simulink model "IndicatorBoard"  (R2023a)
settings: Solver=VariableStepAuto  StartTime=0.0  StopTime=10.0  RelTol=1e-3
libraries: simulink x2
settings Model: Creator=lucas  LastModifiedBy=lucas

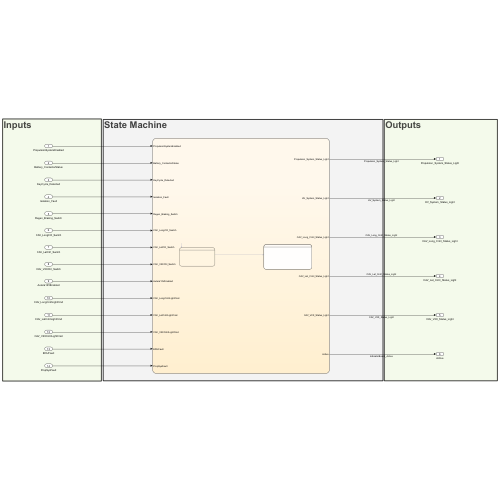
[thumbnail: Simulink's stored preview of the top-level diagram]
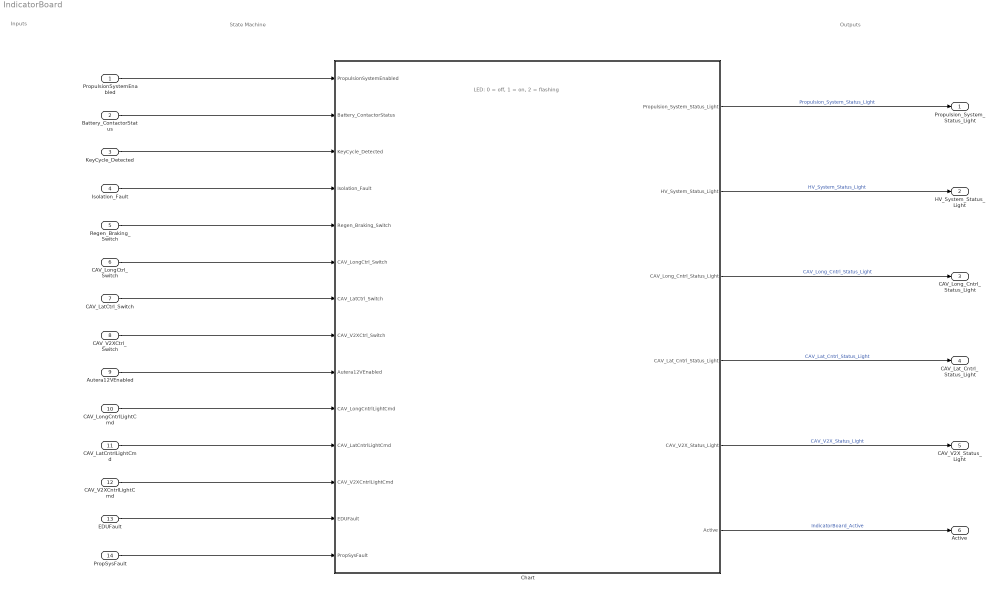
== system IndicatorBoard ==
  note: Inputs
  note: LED: 0 = off, 1 = on, 2 = flashing
  note: Outputs
  note: State Machine
  PropulsionSystemEnabled : Inport
  Battery_ContactorStatus : Inport  Port=2
  KeyCycle_Detected : Inport  Port=3
  Isolation_Fault : Inport  Port=4
  Regen_Braking_Switch : Inport  Port=5
  CAV_LongCtrl_Switch : Inport  Port=6
  CAV_LatCtrl_Switch : Inport  Port=7
  CAV_V2XCtrl_Switch : Inport  Port=8
  Autera12VEnabled : Inport  Port=9
  CAV_LongCntrlLightCmd : Inport  Port=10
  CAV_LatCntrlLightCmd : Inport  Port=11
  CAV_V2XCntrlLightCmd : Inport  Port=12
  EDUFault : Inport  Port=13
  PropSysFault : Inport  Port=14
  Chart : Stateflow chart  TreatAsAtomicUnit=on
  Propulsion_System_Status_Light : Outport
  HV_System_Status_Light : Outport  Port=2
  CAV_Long_Cntrl_Status_Light : Outport  Port=3
  CAV_Lat_Cntrl_Status_Light : Outport  Port=4
  CAV_V2X_Status_Light : Outport  Port=5
  Active : Outport  Port=6
  wires:
  Chart/1(Propulsion_System_Status_Light) -> Propulsion_System_Status_Light/1  "Propulsion_System_Status_Light"
  KeyCycle_Detected/1 -> Chart/3(KeyCycle_Detected)
  Chart/2(HV_System_Status_Light) -> HV_System_Status_Light/1  "HV_System_Status_Light"
  Chart/5(CAV_V2X_Status_Light) -> CAV_V2X_Status_Light/1  "CAV_V2X_Status_Light"
  PropulsionSystemEnabled/1 -> Chart/1(PropulsionSystemEnabled)
  Chart/4(CAV_Lat_Cntrl_Status_Light) -> CAV_Lat_Cntrl_Status_Light/1  "CAV_Lat_Cntrl_Status_Light"
  Chart/3(CAV_Long_Cntrl_Status_Light) -> CAV_Long_Cntrl_Status_Light/1  "CAV_Long_Cntrl_Status_Light"
  Battery_ContactorStatus/1 -> Chart/2(Battery_ContactorStatus)
  Autera12VEnabled/1 -> Chart/9(Autera12VEnabled)
  Isolation_Fault/1 -> Chart/4(Isolation_Fault)
  Regen_Braking_Switch/1 -> Chart/5(Regen_Braking_Switch)
  CAV_LongCtrl_Switch/1 -> Chart/6(CAV_LongCtrl_Switch)
  CAV_LatCtrl_Switch/1 -> Chart/7(CAV_LatCtrl_Switch)
  CAV_V2XCtrl_Switch/1 -> Chart/8(CAV_V2XCtrl_Switch)
  CAV_LongCntrlLightCmd/1 -> Chart/10(CAV_LongCntrlLightCmd)
  EDUFault/1 -> Chart/13(EDUFault)
  CAV_LatCntrlLightCmd/1 -> Chart/11(CAV_LatCntrlLightCmd)
  CAV_V2XCntrlLightCmd/1 -> Chart/12(CAV_V2XCntrlLightCmd)
  PropSysFault/1 -> Chart/14(PropSysFault)
  Chart/6(Active) -> Active/1  "IndicatorBoard_Active"

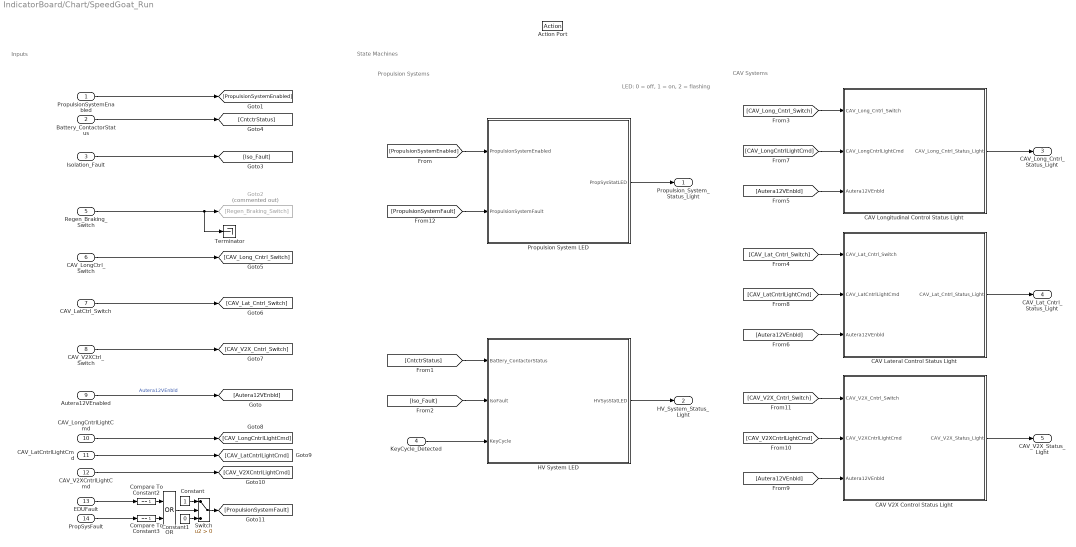
== system IndicatorBoard/Chart/SpeedGoat_Run ==
  note: LED: 0 = off, 1 = on, 2 = flashing
  note: Inputs
  note: State Machines
  note: Propulsion Systems
  note: CAV Systems
  PropulsionSystemEnabled : Inport
  Battery_ContactorStatus : Inport  Port=2
  Isolation_Fault : Inport  Port=3
  KeyCycle_Detected : Inport  Port=4
  Regen_Braking_Switch : Inport  Port=5
  CAV_LongCtrl_Switch : Inport  Port=6
  CAV_LatCtrl_Switch : Inport  Port=7
  CAV_V2XCtrl_Switch : Inport  Port=8
  Autera12VEnabled : Inport  Port=9
  CAV_LongCntrlLightCmd : Inport  Port=10
  CAV_LatCntrlLightCmd : Inport  Port=11
  CAV_V2XCntrlLightCmd : Inport  Port=12
  EDUFault : Inport  Port=13
  PropSysFault : Inport  Port=14
  Action Port : ActionPort
      settings: CopyFcn=Stateflow.SLINSF.SimulinkMan.removeBlockPreDeleteFcn  PreDeleteFcn=Stateflow.SLINSF.SimulinkMan.unsafePredeleteFcn
  CAV Lateral Control Status Light : Stateflow chart  TreatAsAtomicUnit=on
  CAV Longitudinal Control Status Light : Stateflow chart  TreatAsAtomicUnit=on
  CAV V2X Control Status Light : Stateflow chart  TreatAsAtomicUnit=on
  Compare To Constant2 : simulink/Logic and Bit Operations/Compare To Constant  relop===  const=1  OutDataTypeStr=boolean
  Compare To Constant3 : simulink/Logic and Bit Operations/Compare To Constant  relop===  const=1  OutDataTypeStr=boolean
  Constant : Constant
  Constant1 : Constant  Value=0
  Goto2 : Goto  Commented=on  GotoTag=Regen_Braking_Switch
  HV System LED : Stateflow chart  TreatAsAtomicUnit=on
  OR : Logic  Operator=OR  AllPortsSameDT=off  OutDataTypeStr=boolean
  Propulsion System LED : Stateflow chart  TreatAsAtomicUnit=on
  Switch : Switch  Criteria=u2 > Threshold  SaturateOnIntegerOverflow=off  InputSameDT=off
  Terminator : Terminator
  Propulsion_System_Status_Light : Outport
  HV_System_Status_Light : Outport  Port=2
  CAV_Long_Cntrl_Status_Light : Outport  Port=3
  CAV_Lat_Cntrl_Status_Light : Outport  Port=4
  CAV_V2X_Status_Light : Outport  Port=5
  wires:
  KeyCycle_Detected/1 -> HV System LED/3(KeyCycle)
  CAV V2X Control Status Light/1(CAV_V2X_Status_Light) -> CAV_V2X_Status_Light/1
  Constant1/1 -> Switch/3
  Constant/1 -> Switch/1
  Switch/1 -> [PropulsionSystemFault]
  [PropulsionSystemFault] -> Propulsion System LED/2(PropulsionSystemFault)
  OR/1 -> Switch/2
  Compare To Constant3/1 -> OR/2
  Compare To Constant2/1 -> OR/1
  PropSysFault/1 -> Compare To Constant3/1
  EDUFault/1 -> Compare To Constant2/1
  [CAV_V2X_Cntrl_Switch] -> CAV V2X Control Status Light/1(CAV_V2X_Cntrl_Switch)
  [CAV_V2XCntrlLightCmd] -> CAV V2X Control Status Light/2(CAV_V2XCntrlLightCmd)
  [Autera12VEnbld] -> CAV V2X Control Status Light/3(Autera12VEnbld)
  [Autera12VEnbld] -> CAV Lateral Control Status Light/3(Autera12VEnbld)
  [CAV_LatCntrlLightCmd] -> CAV Lateral Control Status Light/2(CAV_LatCntrlLightCmd)
  [CAV_Lat_Cntrl_Switch] -> CAV Lateral Control Status Light/1(CAV_Lat_Cntrl_Switch)
  [CAV_LongCntrlLightCmd] -> CAV Longitudinal Control Status Light/2(CAV_LongCntrlLightCmd)
  CAV_V2XCntrlLightCmd/1 -> [CAV_V2XCntrlLightCmd]
  CAV_LatCntrlLightCmd/1 -> [CAV_LatCntrlLightCmd]
  CAV_LongCntrlLightCmd/1 -> [CAV_LongCntrlLightCmd]
  [CAV_Long_Cntrl_Switch] -> CAV Longitudinal Control Status Light/1(CAV_Long_Cntrl_Switch)
  [Autera12VEnbld] -> CAV Longitudinal Control Status Light/3(Autera12VEnbld)
  CAV Longitudinal Control Status Light/1(CAV_Long_Cntrl_Status_Light) -> CAV_Long_Cntrl_Status_Light/1
  CAV Lateral Control Status Light/1(CAV_Lat_Cntrl_Status_Light) -> CAV_Lat_Cntrl_Status_Light/1
  HV System LED/1(HVSysStatLED) -> HV_System_Status_Light/1
  Propulsion System LED/1(PropSysStatLED) -> Propulsion_System_Status_Light/1
  [Iso_Fault] -> HV System LED/2(IsoFault)
  [CntctrStatus] -> HV System LED/1(Battery_ContactorStatus)
  [PropulsionSystemEnabled] -> Propulsion System LED/1(PropulsionSystemEnabled)
  CAV_V2XCtrl_Switch/1 -> [CAV_V2X_Cntrl_Switch]
  CAV_LatCtrl_Switch/1 -> [CAV_Lat_Cntrl_Switch]
  CAV_LongCtrl_Switch/1 -> [CAV_Long_Cntrl_Switch]
  Regen_Braking_Switch/1 -> Terminator/1, Goto2/1
  Autera12VEnabled/1 -> [Autera12VEnbld]  "Autera12VEnbld"
  Battery_ContactorStatus/1 -> [CntctrStatus]
  PropulsionSystemEnabled/1 -> [PropulsionSystemEnabled]
  Isolation_Fault/1 -> [Iso_Fault]

== stateflow chart IndicatorBoard/Chart ==
  state SpeedGoat_Run
  state SpeedGoat_Startup
    state On_Off [group]
      state All_Off
        entry:
        CAV_Lat_Cntrl_Status_Light = 0;
        CAV_Long_Cntrl_Status_Light = 0;
        CAV_V2X_Status_Light = 0;
        HV_System_Status_Light = 0;
        Propulsion_System_Status_Light = 0;
      state All_On
        entry:
        CAV_Lat_Cntrl_Status_Light = 1;
        CAV_Long_Cntrl_Status_Light = 1;
        CAV_V2X_Status_Light = 1;
        HV_System_Status_Light = 1;
        Propulsion_System_Status_Light = 1;
      state All_Off1
        entry:
        CAV_Lat_Cntrl_Status_Light = 0;
        CAV_Long_Cntrl_Status_Light = 0;
        CAV_V2X_Status_Light = 0;
        HV_System_Status_Light = 0;
        Propulsion_System_Status_Light = 0;
      state All_On1
        entry:
        CAV_Lat_Cntrl_Status_Light = 1;
        CAV_Long_Cntrl_Status_Light = 1;
        CAV_V2X_Status_Light = 1;
        HV_System_Status_Light = 1;
        Propulsion_System_Status_Light = 1;
      state All_Off2
        entry:
        CAV_Lat_Cntrl_Status_Light = 0;
        CAV_Long_Cntrl_Status_Light = 0;
        CAV_V2X_Status_Light = 0;
        HV_System_Status_Light = 0;
        Propulsion_System_Status_Light = 0;
      state All_On2
        entry:
        CAV_Lat_Cntrl_Status_Light = 1;
        CAV_Long_Cntrl_Status_Light = 1;
        CAV_V2X_Status_Light = 1;
        HV_System_Status_Light = 1;
        Propulsion_System_Status_Light = 1;
      state All_Off3
        entry:
        CAV_Lat_Cntrl_Status_Light = 0;
        CAV_Long_Cntrl_Status_Light = 0;
        CAV_V2X_Status_Light = 0;
        HV_System_Status_Light = 0;
        Propulsion_System_Status_Light = 0;
      (default) -> All_Off
      All_On -> All_Off1 : after(0.2,sec)
      All_Off1 -> All_On1 : after(0.2,sec)
      All_On1 -> All_Off2 : after(0.2,sec)
      All_On2 -> All_Off3 : after(0.2,sec)
      All_Off2 -> All_On2 : after(0.2,sec)
      All_Off -> All_On : after(0.2,sec)
    state Side_To_Side [group]
      state LED2_2
        entry:
        CAV_Lat_Cntrl_Status_Light = 0;
        CAV_Long_Cntrl_Status_Light = 0;
        CAV_V2X_Status_Light = 0;
        HV_System_Status_Light = 1;
        Propulsion_System_Status_Light = 0;
      state LED1_1
        entry:
        CAV_Lat_Cntrl_Status_Light = 0;
        CAV_Long_Cntrl_Status_Light = 0;
        CAV_V2X_Status_Light = 0;
        HV_System_Status_Light = 0;
        Propulsion_System_Status_Light = 1;
      state LED1_2
        entry:
        CAV_Lat_Cntrl_Status_Light = 0;
        CAV_Long_Cntrl_Status_Light = 0;
        CAV_V2X_Status_Light = 0;
        HV_System_Status_Light = 0;
        Propulsion_System_Status_Light = 1;
      state LED1_3
        entry:
        CAV_Lat_Cntrl_Status_Light = 0;
        CAV_Long_Cntrl_Status_Light = 0;
        CAV_V2X_Status_Light = 0;
        HV_System_Status_Light = 0;
        Propulsion_System_Status_Light = 1;
      state LED1_4
        entry:
        CAV_Lat_Cntrl_Status_Light = 0;
        CAV_Long_Cntrl_Status_Light = 0;
        CAV_V2X_Status_Light = 0;
        HV_System_Status_Light = 0;
        Propulsion_System_Status_Light = 1;
      state LED2_6
        entry:
        CAV_Lat_Cntrl_Status_Light = 0;
        CAV_Long_Cntrl_Status_Light = 0;
        CAV_V2X_Status_Light = 0;
        HV_System_Status_Light = 1;
        Propulsion_System_Status_Light = 0;
      state LED2_4
        entry:
        CAV_Lat_Cntrl_Status_Light = 0;
        CAV_Long_Cntrl_Status_Light = 0;
        CAV_V2X_Status_Light = 0;
        HV_System_Status_Light = 1;
        Propulsion_System_Status_Light = 0;
      state LED3_2
        entry:
        CAV_Lat_Cntrl_Status_Light = 0;
        CAV_Long_Cntrl_Status_Light = 1;
        CAV_V2X_Status_Light = 0;
        HV_System_Status_Light = 0;
        Propulsion_System_Status_Light = 0;
      state LED2_5
        entry:
        CAV_Lat_Cntrl_Status_Light = 0;
        CAV_Long_Cntrl_Status_Light = 0;
        CAV_V2X_Status_Light = 0;
        HV_System_Status_Light = 1;
        Propulsion_System_Status_Light = 0;
      state LED3_6
        entry:
        CAV_Lat_Cntrl_Status_Light = 0;
        CAV_Long_Cntrl_Status_Light = 1;
        CAV_V2X_Status_Light = 0;
        HV_System_Status_Light = 0;
        Propulsion_System_Status_Light = 0;
      state LED2_1
        entry:
        CAV_Lat_Cntrl_Status_Light = 0;
        CAV_Long_Cntrl_Status_Light = 0;
        CAV_V2X_Status_Light = 0;
        HV_System_Status_Light = 1;
        Propulsion_System_Status_Light = 0;
      state LED2_3
        entry:
        CAV_Lat_Cntrl_Status_Light = 0;
        CAV_Long_Cntrl_Status_Light = 0;
        CAV_V2X_Status_Light = 0;
        HV_System_Status_Light = 1;
        Propulsion_System_Status_Light = 0;
      state LED3_4
        entry:
        CAV_Lat_Cntrl_Status_Light = 0;
        CAV_Long_Cntrl_Status_Light = 1;
        CAV_V2X_Status_Light = 0;
        HV_System_Status_Light = 0;
        Propulsion_System_Status_Light = 0;
      state LED4_6
        entry:
        CAV_Lat_Cntrl_Status_Light = 1;
        CAV_Long_Cntrl_Status_Light = 0;
        CAV_V2X_Status_Light = 0;
        HV_System_Status_Light = 0;
        Propulsion_System_Status_Light = 0;
      state LED3_5
        entry:
        CAV_Lat_Cntrl_Status_Light = 0;
        CAV_Long_Cntrl_Status_Light = 1;
        CAV_V2X_Status_Light = 0;
        HV_System_Status_Light = 0;
        Propulsion_System_Status_Light = 0;
      state LED4_2
        entry:
        CAV_Lat_Cntrl_Status_Light = 1;
        CAV_Long_Cntrl_Status_Light = 0;
        CAV_V2X_Status_Light = 0;
        HV_System_Status_Light = 0;
        Propulsion_System_Status_Light = 0;
      state LED4_4
        entry:
        CAV_Lat_Cntrl_Status_Light = 1;
        CAV_Long_Cntrl_Status_Light = 0;
        CAV_V2X_Status_Light = 0;
        HV_System_Status_Light = 0;
        Propulsion_System_Status_Light = 0;
      state LED3_3
        entry:
        CAV_Lat_Cntrl_Status_Light = 0;
        CAV_Long_Cntrl_Status_Light = 1;
        CAV_V2X_Status_Light = 0;
        HV_System_Status_Light = 0;
        Propulsion_System_Status_Light = 0;
      state LED3_1
        entry:
        CAV_Lat_Cntrl_Status_Light = 0;
        CAV_Long_Cntrl_Status_Light = 1;
        CAV_V2X_Status_Light = 0;
        HV_System_Status_Light = 0;
        Propulsion_System_Status_Light = 0;
      state LED5_3
        entry:
        CAV_Lat_Cntrl_Status_Light = 0;
        CAV_Long_Cntrl_Status_Light = 0;
        CAV_V2X_Status_Light = 1;
        HV_System_Status_Light = 0;
        Propulsion_System_Status_Light = 0;
      state LED4_5
        entry:
        CAV_Lat_Cntrl_Status_Light = 1;
        CAV_Long_Cntrl_Status_Light = 0;
        CAV_V2X_Status_Light = 0;
        HV_System_Status_Light = 0;
        Propulsion_System_Status_Light = 0;
      state LED5_1
        entry:
        CAV_Lat_Cntrl_Status_Light = 0;
        CAV_Long_Cntrl_Status_Light = 0;
        CAV_V2X_Status_Light = 1;
        HV_System_Status_Light = 0;
        Propulsion_System_Status_Light = 0;
      state LED5_2
        entry:
        CAV_Lat_Cntrl_Status_Light = 0;
        CAV_Long_Cntrl_Status_Light = 0;
        CAV_V2X_Status_Light = 1;
        HV_System_Status_Light = 0;
        Propulsion_System_Status_Light = 0;
      state LED4_3
        entry:
        CAV_Lat_Cntrl_Status_Light = 1;
        CAV_Long_Cntrl_Status_Light = 0;
        CAV_V2X_Status_Light = 0;
        HV_System_Status_Light = 0;
        Propulsion_System_Status_Light = 0;
      state LED4_1
        entry:
        CAV_Lat_Cntrl_Status_Light = 1;
        CAV_Long_Cntrl_Status_Light = 0;
        CAV_V2X_Status_Light = 0;
        HV_System_Status_Light = 0;
        Propulsion_System_Status_Light = 0;
      LED2_6 -> LED1_4 : after(0.1,sec)
      LED2_2 -> LED1_2 : after(0.1,sec)
      LED2_4 -> LED1_3 : after(0.1,sec)
      LED3_2 -> LED2_2 : after(0.1,sec)
      LED1_1 -> LED2_1 : after(0.1,sec)
      LED1_2 -> LED2_3 : after(0.1,sec)
      LED3_6 -> LED2_6 : after(0.1,sec)
      LED1_3 -> LED2_5 : after(0.1,sec)
      LED3_4 -> LED2_4 : after(0.1,sec)
      LED4_6 -> LED3_6 : after(0.1,sec)
      LED2_5 -> LED3_5 : after(0.1,sec)
      LED4_2 -> LED3_2 : after(0.1,sec)
      LED2_1 -> LED3_1 : after(0.1,sec)
      LED2_3 -> LED3_3 : after(0.1,sec)
      LED4_4 -> LED3_4 : after(0.1,sec)
      LED5_3 -> LED4_6 : after(0.1,sec)
      LED3_5 -> LED4_5 : after(0.1,sec)
      LED5_1 -> LED4_2 : after(0.1,sec)
      LED5_2 -> LED4_4 : after(0.1,sec)
      LED3_3 -> LED4_3 : after(0.1,sec)
      LED3_1 -> LED4_1 : after(0.1,sec)
      LED4_3 -> LED5_2 : after(0.1,sec)
      LED4_5 -> LED5_3 : after(0.1,sec)
      LED4_1 -> LED5_1 : after(0.1,sec)
    LED1_4 -> All_Off : after(0.1,sec)
    All_Off3 -> LED1_1 : after(0.1,sec)
  (default) -> SpeedGoat_Startup : {Active = 0;}
  SpeedGoat_Startup -> SpeedGoat_Run : [after(10,sec) || Isolation_Fault == 1]{Active = 1;}
  data: sf_internal_action_state_placeholder_data local double size=1 =0; PropulsionSystemEnabled input; Battery_ContactorStatus input; KeyCycle_Detected input; Propulsion_System_Status_Light output; HV_System_Status_Light output; CAV_Long_Cntrl_Status_Light output; CAV_Lat_Cntrl_Status_Light output; CAV_V2X_Status_Light output; Isolation_Fault input; Regen_Braking_Switch input; CAV_LongCtrl_Switch input; CAV_LatCtrl_Switch input; CAV_V2XCtrl_Switch input; Autera12VEnabled input; CAV_LongCntrlLightCmd input; CAV_LatCntrlLightCmd input; CAV_V2XCntrlLightCmd input; EDUFault input; PropSysFault input; Active output

== stateflow chart IndicatorBoard/Chart/SpeedGoat_Run/CAV Longitudinal Control Status Light ==
  state Off
    during:
    CAV_Long_Cntrl_Status_Light = 0;
  state On
    during:
    CAV_Long_Cntrl_Status_Light = 1;
  state Flashing
    during:
    CAV_Long_Cntrl_Status_Light = 2;
  (default) -> Off
  Off -> On [order 1] : [Autera12VEnbld == 1 && CAV_Long_Cntrl_Switch == 1 && CAV_LongCntrlLightCmd == 1]
  On -> Off [order 1] : [Autera12VEnbld == 0 || CAV_LongCntrlLightCmd == 0 || CAV_Long_Cntrl_Switch == 0]
  Flashing -> Off [order 2] : [Autera12VEnbld == 0 || ...
      | CAV_LongCntrlLightCmd == 0 || ...
      | CAV_Long_Cntrl_Switch == 0]
  Off -> Flashing [order 2] : [Autera12VEnbld == 1 && ...
      |  CAV_Long_Cntrl_Switch == 1 && ...
      | CAV_LongCntrlLightCmd == 2]
  Flashing -> On [order 1] : [Autera12VEnbld == 1 && ...
      | CAV_Long_Cntrl_Switch == 1 && ...
      | CAV_LongCntrlLightCmd == 1]
  On -> Flashing [order 2] : [Autera12VEnbld == 1 && ...
      |  CAV_Long_Cntrl_Switch == 1 && ...
      | CAV_LongCntrlLightCmd == 2]
  data: CAV_Long_Cntrl_Switch input; CAV_LongCntrlLightCmd input; CAV_Long_Cntrl_Status_Light output; Autera12VEnbld input

== stateflow chart IndicatorBoard/Chart/SpeedGoat_Run/CAV Lateral Control Status Light ==
  state Off
    during:
    CAV_Lat_Cntrl_Status_Light = 0;
  state On
    during:
    CAV_Lat_Cntrl_Status_Light = 1;
  state Flashing
    during:
    CAV_Lat_Cntrl_Status_Light = 2;
  (default) -> Off
  Off -> On [order 1] : [Autera12VEnbld == 1 && CAV_Lat_Cntrl_Switch == 1 && CAV_LatCntrlLightCmd == 1]
  On -> Off [order 1] : [Autera12VEnbld == 0 || CAV_LatCntrlLightCmd == 0 || CAV_Lat_Cntrl_Switch == 0]
  Flashing -> Off [order 2] : [Autera12VEnbld == 0 || ...
      | CAV_LatCntrlLightCmd == 0 || ...
      | CAV_Lat_Cntrl_Switch == 0]
  Off -> Flashing [order 2] : [Autera12VEnbld == 1 && ...
      |  CAV_Lat_Cntrl_Switch == 1 && ...
      | CAV_LatCntrlLightCmd == 2]
  Flashing -> On [order 1] : [Autera12VEnbld == 1 && ...
      | CAV_Lat_Cntrl_Switch == 1 && ...
      | CAV_LatCntrlLightCmd == 1]
  On -> Flashing [order 2] : [Autera12VEnbld == 1 && ...
      |  CAV_Lat_Cntrl_Switch == 1 && ...
      | CAV_LatCntrlLightCmd == 2]
  data: CAV_Lat_Cntrl_Switch input; CAV_LatCntrlLightCmd input; CAV_Lat_Cntrl_Status_Light output; Autera12VEnbld input

== stateflow chart IndicatorBoard/Chart/SpeedGoat_Run/HV System LED ==
  state Off
    during: HVSysStatLED = 0;
  state On
    during: HVSysStatLED = 1;
  state Flashing
    during: HVSysStatLED = 2;
  (default) -> Off
  Off -> On [order 1] : [(Battery_ContactorStatus == 2 && (IsoFault == 0))]
  On -> Off [order 1] : [(Battery_ContactorStatus == 0) && (IsoFault == 0)]
  Flashing -> Off [order 2] : [(Battery_ContactorStatus == 0) && (IsoFault == 0)&& KeyCycle ==1]
  Off -> Flashing [order 2] : [IsoFault == 1]
  Flashing -> On [order 1] : [(Battery_ContactorStatus == 2) && (IsoFault == 0) && KeyCycle ==1]
  On -> Flashing [order 2] : [IsoFault == 1]
  data: Battery_ContactorStatus input; HVSysStatLED output; IsoFault input; KeyCycle input

== stateflow chart IndicatorBoard/Chart/SpeedGoat_Run/Propulsion System LED ==
  state Off
    during: PropSysStatLED = 0;
  state On
    during: PropSysStatLED = 1;
  state Flashing
    during: PropSysStatLED = 2;
  (default) -> Off
  Off -> On [order 1] : [(PropulsionSystemEnabled == 1 && (PropulsionSystemFault == 0))]
  On -> Off [order 1] : [(PropulsionSystemEnabled == 0) && (PropulsionSystemFault == 0)]
  Flashing -> Off [order 2] : [(PropulsionSystemEnabled == 0) && (PropulsionSystemFault == 0)]
  Off -> Flashing [order 2] : [PropulsionSystemFault == 1]
  Flashing -> On [order 1] : [(PropulsionSystemEnabled == 1) && (PropulsionSystemFault == 0)]
  On -> Flashing [order 2] : [PropulsionSystemFault == 1]
  data: PropulsionSystemEnabled input; PropSysStatLED output; PropulsionSystemFault input

== stateflow chart IndicatorBoard/Chart/SpeedGoat_Run/CAV V2X Control Status Light ==
  state Off
    during:
    CAV_V2X_Status_Light = 0;
  state On
    during:
    CAV_V2X_Status_Light = 1;
  state Flashing
    during:
    CAV_V2X_Status_Light = 2;
  (default) -> Off
  Off -> On [order 1] : [Autera12VEnbld == 1 && CAV_V2X_Cntrl_Switch == 1 && CAV_V2XCntrlLightCmd == 1]
  On -> Off [order 1] : [Autera12VEnbld == 0 || CAV_V2XCntrlLightCmd == 0 || CAV_V2X_Cntrl_Switch == 0]
  Flashing -> Off [order 2] : [Autera12VEnbld == 0 || ...
      | CAV_V2XCntrlLightCmd == 0 || ...
      | CAV_V2X_Cntrl_Switch == 0]
  Off -> Flashing [order 2] : [Autera12VEnbld == 1 && ...
      |  CAV_V2X_Cntrl_Switch == 1 && ...
      | CAV_V2XCntrlLightCmd == 2]
  Flashing -> On [order 1] : [Autera12VEnbld == 1 && ...
      | CAV_V2X_Cntrl_Switch == 1 && ...
      | CAV_V2XCntrlLightCmd == 1]
  On -> Flashing [order 2] : [Autera12VEnbld == 1 && ...
      |  CAV_V2X_Cntrl_Switch == 1 && ...
      | CAV_V2XCntrlLightCmd == 2]
  data: CAV_V2X_Cntrl_Switch input; CAV_V2XCntrlLightCmd input; CAV_V2X_Status_Light output; Autera12VEnbld input
